simulink model "three_ph_SCR"  (R2018a)
settings: Solver=VariableStepAuto  StartTime=-0.04  StopTime=0.02  MaxStep=1e-5  RelTol=1e-3
undefined symbols (not defined in the file or in its folder): D1, lagging, pulse
libraries: powerlib x14, powerlib_meascontrol x1, simulink x1
settings Model: Creator=pdb  LastModifiedBy=pdb
settings DebuggingCC: UnconnectedOutputMsg=none

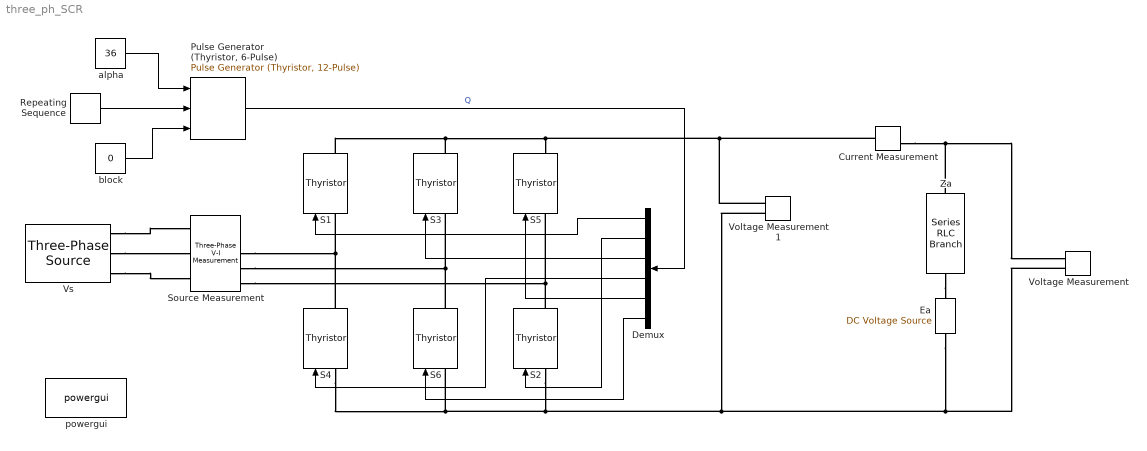
== system three_ph_SCR ==
  Current Measurement : powerlib/Measurements/Current Measurement  PhasorSimulation=off  OutputType=Complex  PSBequivalent=0
  Demux : Demux  Outputs=6
  Ea : powerlib/Electrical Sources/DC Voltage Source  Amplitude=202  Measurements=None
  "Pulse Generator (Thyristor, 6-Pulse)" : powerlib_meascontrol/Pulse & Signal Generators/Pulse Generator (Thyristor, 12-Pulse)  GenType=6-pulse  Delta=D1 (lagging)  pwidth=15  Double_Pulse=on  Ts=0
      settings: SourceProductName=Simscape Power Systems  SourceProductBaseCode=PS
  Repeating Sequence : simulink/Sources/Repeating Sequence  rep_seq_t=[0 1/50]  rep_seq_y=[0 2*pi]
  S{1..6} (6 alike) : powerlib/Power Electronics/Thyristor  Ron=0.001  Lon=0  Vf=1.5  IC=0  Rs=inf  Cs=0  Measurements=on
  Source Measurement : powerlib/Measurements/Three-Phase V-I Measurement  VoltageMeasurement=phase-to-ground  SetLabelV=off  LabelV=Vabc  Vpu=off  VpuLL=off  CurrentMeasurement=yes  SetLabelI=off  LabelI=Iabc  Ipu=off  Pbase=100e6  Vbase=500e3  OutputType=Complex  PhasorSimulation=off  PSBequivalent=0
  Voltage Measurement : powerlib/Measurements/Voltage Measurement  PhasorSimulation=off  OutputType=Complex  PSBequivalent=0
  Voltage Measurement1 : powerlib/Measurements/Voltage Measurement  PhasorSimulation=off  OutputType=Complex  PSBequivalent=0
  Vs : powerlib/Electrical Sources/Three-Phase Source  InternalConnection=Yg  VoltagePhases=off  Voltage=120*sqrt(3)  PhaseAngle=0  Voltage_phases=[25e3 25e3 25e3]/sqrt(3)  PhaseAngles_phases=[0 -120 +120]  Frequency=50  NonIdealSource=on  SpecifyImpedance=off  Resistance=0.05  Inductance=1.8e-4  ShortCircuitLevel=sqrt(3)*220*20000  BaseVoltage=120*sqrt(3)  XRratio=0.1  BusType=swing  Pref=10e3  Qref=0  Prefabc=[10e3, 10e3, 10e3]  Qrefabc=[0, 0, 0]  Qmin=-inf  Qmax=inf
  Za : powerlib/Elements/Series RLC Branch  LConnTagsString=__new0  RConnTagsString=__new0  BranchType=RL  Resistance=0.8  Inductance=0.0125  SetiL0=off  InitialCurrent=0  Capacitance=1e-6  Setx0=off  InitialVoltage=0  Measurements=None
  alpha : Constant  Value=36
  block : Constant  Value=0
  powergui : powerlib/powergui  Priority=1  SimulationMode=Continuous  SampleTime=50e-6  frequency=60  Iterations=50  frequencyindice=0  Pbase=100e6  ErrMax=1e-4  UnitsV=kV  UnitsW=MW  buscounter=0  FunctionMessages=off  echomessages=off  EnableUseOfTLC=off  CurrentSourceSwitches=off  DisableSnubberDevices=off  DisableRonSwitches=off  DisableVfSwitches=off  DisplayEquations=off  SolverType=Tustin/Backward Euler (TBE)  Interpol=off  ExternalGateDelay=off  methode=off  Ts=100  x0status=blocks  SPID=on  SwTol=0  HookPort=off  RestoreLinks=warning  ResistiveCurrentMeasurement=off  Frange=[0:2:500]  Ylog=off  Xlog=on  ShowGrid=off  save=off  variable=ZData  structure=0  ZoomFFT=off  StartTime=0.0  cycles=1  DisplayStyle=1  fundamental=60  FreqAxis=off  MaxFrequency=1000  frequencyindicesteady=1  RmsSteady=1  display=off
  wires:
  "Pulse Generator (Thyristor, 6-Pulse)"/1 -> Demux/1  "Q"
  alpha/1 -> "Pulse Generator (Thyristor, 6-Pulse)"/1
  Repeating Sequence/1 -> "Pulse Generator (Thyristor, 6-Pulse)"/2
  Demux/1 -> S1/1
  Demux/2 -> S2/1
  Demux/3 -> S3/1
  Demux/5 -> S5/1
  Demux/4 -> S4/1
  Demux/6 -> S6/1
  block/1 -> "Pulse Generator (Thyristor, 6-Pulse)"/3
  connections:
  Vs/RConn1 -- Source Measurement/LConn1
  Vs/RConn2 -- Source Measurement/LConn2
  Vs/RConn3 -- Source Measurement/LConn3
  S4/RConn1 -- Source Measurement/RConn1 -- S1/LConn1
  S6/RConn1 -- Source Measurement/RConn2 -- S3/LConn1
  S2/RConn1 -- Source Measurement/RConn3 -- S5/LConn1
  S1/RConn1 -- S3/RConn1 -- Current Measurement/LConn1 -- Voltage Measurement1/LConn1 -- S5/RConn1
  S4/LConn1 -- Voltage Measurement/LConn2 -- Ea/LConn1 -- Voltage Measurement1/LConn2 -- S2/LConn1 -- S6/LConn1
  Current Measurement/RConn1 -- Za/LConn1 -- Voltage Measurement/LConn1
  Za/RConn1 -- Ea/RConn1
